simulink model "example"  (R2018a)
settings: Solver=FixedStepAuto  StartTime=0.0  StopTime=data.T_end  FixedStep=1e-4  RelTol=1e-3
InitFcn:
  | run initSim
StopFcn:
  | run endSim
undefined symbols (not defined in the file or in its folder): data
libraries: simulink x2
settings Model: Creator=Matteo Ragni  LastModifiedBy=nirva

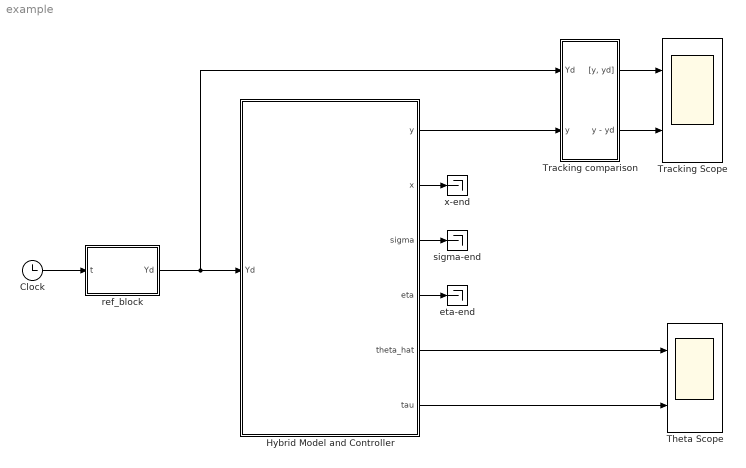
== system example ==
  Clock : Clock
  Hybrid Model and Controller : Subsystem
  Theta Scope : Scope  NumInputPorts=2
  Tracking Scope : Scope  NumInputPorts=2
  Tracking comparison : Subsystem
  eta-end : Terminator
  ref_block : MATLAB Function  TreatAsAtomicUnit=on
  sigma-end : Terminator
  x-end : Terminator
  wires:
  Clock/1 -> ref_block/1(t)
  ref_block/1(Yd) -> Tracking comparison/1(Yd), Hybrid Model and Controller/1(Yd)
  Hybrid Model and Controller/1(y) -> Tracking comparison/2(y)
  Tracking comparison/1("[y, yd]") -> Tracking Scope/1
  Tracking comparison/2(y - yd) -> Tracking Scope/2
  Hybrid Model and Controller/2(x) -> x-end/1
  Hybrid Model and Controller/3(sigma) -> sigma-end/1
  Hybrid Model and Controller/4(eta) -> eta-end/1
  Hybrid Model and Controller/5(theta_hat) -> Theta Scope/1
  Hybrid Model and Controller/6(tau) -> Theta Scope/2

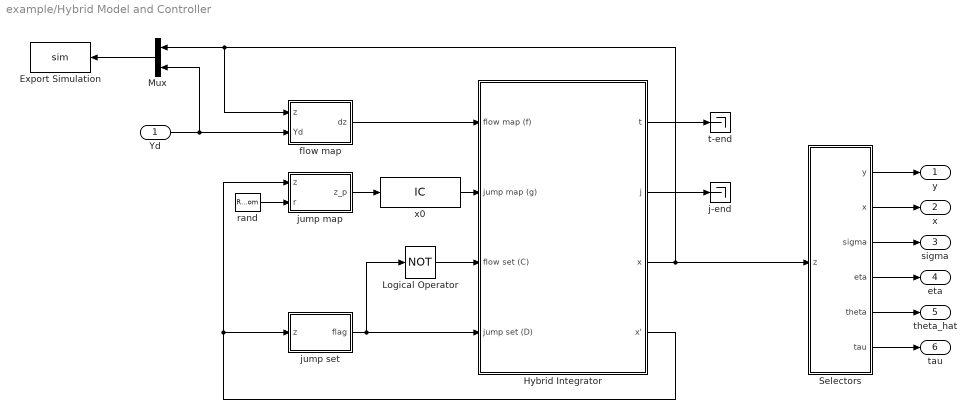
== system example/Hybrid Model and Controller ==
  Yd : Inport
  Export Simulation : ToWorkspace  VariableName=sim  SampleTime=-1
  Hybrid Integrator : Subsystem
  Logical Operator : Logic  Operator=NOT  AllPortsSameDT=off  OutDataTypeStr=boolean
  Mux : Mux  Inputs=2
  Selectors : Subsystem
  flow map : MATLAB Function  TreatAsAtomicUnit=on
  j-end : Terminator
  jump map : MATLAB Function  Priority=2  TreatAsAtomicUnit=on
  jump set : MATLAB Function  TreatAsAtomicUnit=on
  rand : UniformRandomNumber  Minimum=0  SampleTime=0.001
  t-end : Terminator
  x0 : InitialCondition  Value=data.ics
  y : Outport
  x : Outport  Port=2
  sigma : Outport  Port=3
  eta : Outport  Port=4
  theta_hat : Outport  Port=5
  tau : Outport  Port=6
  wires:
  Yd/1 -> Mux/2, flow map/2(Yd)
  Hybrid Integrator/1(t) -> t-end/1
  Hybrid Integrator/2(j) -> j-end/1
  Hybrid Integrator/4(x') -> jump map/1(z), jump set/1(z)
  jump set/1(flag) -> Hybrid Integrator/4(jump set (D)), Logical Operator/1
  Hybrid Integrator/3(x) -> Selectors/1(z), flow map/1(z), Mux/1
  flow map/1(dz) -> Hybrid Integrator/1(flow map (f))
  jump map/1(z_p) -> x0/1
  x0/1 -> Hybrid Integrator/2(jump map (g))
  Logical Operator/1 -> Hybrid Integrator/3(flow set (C))
  rand/1 -> jump map/2(r)
  Selectors/1(y) -> y/1
  Selectors/2(x) -> x/1
  Selectors/3(sigma) -> sigma/1
  Selectors/4(eta) -> eta/1
  Selectors/5(theta) -> theta_hat/1
  Selectors/6(tau) -> tau/1
  Mux/1 -> Export Simulation/1

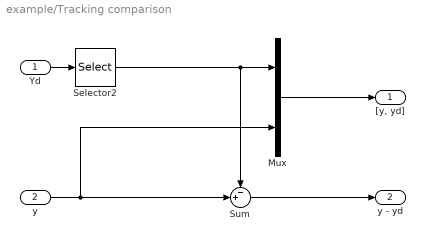
== system example/Tracking comparison ==
  Yd : Inport
  y : Inport  Port=2
  Mux : Mux  Inputs=2
  Selector2 : Selector  InputPortWidth=data.theta_n  IndexOptions=Index vector (dialog)  Indices=[1]  OutputSizes=1
  Sum : Sum  Inputs=-+|
  "[y, yd]" : Outport
  y - yd : Outport  Port=2
  wires:
  Yd/1 -> Selector2/1
  Selector2/1 -> Sum/1, Mux/1
  Mux/1 -> "[y, yd]"/1
  Sum/1 -> y - yd/1
  y/1 -> Mux/2, Sum/2

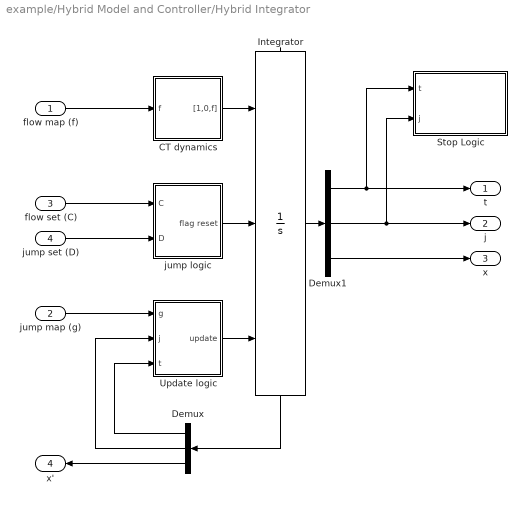
== system example/Hybrid Model and Controller/Hybrid Integrator ==
  flow map (f) : Inport
  jump map (g) : Inport  Port=2
  flow set (C) : Inport  Port=3
  jump set (D) : Inport  Port=4
  CT dynamics : Subsystem
  Demux : Demux  Outputs=[1 ,1, length(data.ics)]
  Demux1 : Demux  Outputs=[1, 1, length(data.ics)]
  Integrator : Integrator  ExternalReset=level hold  InitialConditionSource=external  ShowStatePort=on  ZeroCross=off
  Stop Logic : Subsystem
  Update logic : Subsystem
  jump logic : Subsystem
  t : Outport
  j : Outport  Port=2
  x : Outport  Port=3
  x' : Outport  Port=4
  wires:
  Integrator/State -> Demux/1
  flow map (f)/1 -> CT dynamics/1(f)
  flow set (C)/1 -> jump logic/1(C)
  CT dynamics/1("[1,0,f]") -> Integrator/1
  jump logic/1(flag reset) -> Integrator/2
  jump set (D)/1 -> jump logic/2(D)
  Update logic/1(update) -> Integrator/3
  Demux/1 -> Update logic/3(t)
  Demux/2 -> Update logic/2(j)
  jump map (g)/1 -> Update logic/1(g)
  Demux/3 -> x'/1
  Integrator/1 -> Demux1/1
  Demux1/1 -> Stop Logic/1(t), t/1
  Demux1/2 -> Stop Logic/2(j), j/1
  Demux1/3 -> x/1

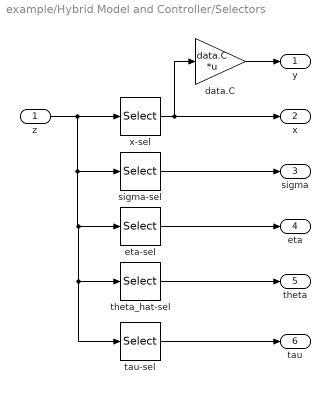
== system example/Hybrid Model and Controller/Selectors ==
  z : Inport
  data.C : Gain  Gain=data.C  Multiplication=Matrix(K*u)
  eta-sel : Selector  InputPortWidth=size(data.ics, 1)  IndexOptions=Index vector (dialog)  Indices=data.index.eta  OutputSizes=1
  sigma-sel : Selector  InputPortWidth=size(data.ics, 1)  IndexOptions=Index vector (dialog)  Indices=data.index.sigma  OutputSizes=1
  tau-sel : Selector  InputPortWidth=size(data.ics, 1)  IndexOptions=Index vector (dialog)  Indices=data.index.tau  OutputSizes=1
  theta_hat-sel : Selector  InputPortWidth=size(data.ics, 1)  IndexOptions=Index vector (dialog)  Indices=data.index.theta_hat  OutputSizes=1
  x-sel : Selector  InputPortWidth=size(data.ics, 1)  IndexOptions=Index vector (dialog)  Indices=data.index.x  OutputSizes=1
  y : Outport
  x : Outport  Port=2
  sigma : Outport  Port=3
  eta : Outport  Port=4
  theta : Outport  Port=5
  tau : Outport  Port=6
  wires:
  z/1 -> tau-sel/1, theta_hat-sel/1, eta-sel/1, sigma-sel/1, x-sel/1
  x-sel/1 -> x/1, data.C/1
  sigma-sel/1 -> sigma/1
  theta_hat-sel/1 -> theta/1
  data.C/1 -> y/1
  tau-sel/1 -> tau/1
  eta-sel/1 -> eta/1

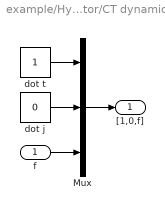
== system example/Hybrid Model and Controller/Hybrid Integrator/CT dynamics ==
  f : Inport
  Mux : Mux  Inputs=3
  dot j : Constant  Value=0
  dot t : Constant
  "[1,0,f]" : Outport
  wires:
  Mux/1 -> "[1,0,f]"/1
  f/1 -> Mux/3
  dot t/1 -> Mux/1
  dot j/1 -> Mux/2

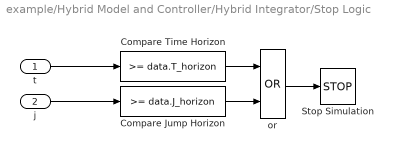
== system example/Hybrid Model and Controller/Hybrid Integrator/Stop Logic ==
  t : Inport
  j : Inport  Port=2
  Compare Jump Horizon : simulink/Logic and Bit Operations/Compare To Constant  relop=>=  const=data.J_horizon  OutDataTypeStr=boolean
  Compare Time Horizon : simulink/Logic and Bit Operations/Compare To Constant  relop=>=  const=data.T_horizon  OutDataTypeStr=boolean
  Stop Simulation : Stop
  or : Logic  Operator=OR  AllPortsSameDT=off  OutDataTypeStr=boolean
  wires:
  Compare Jump Horizon/1 -> or/2
  t/1 -> Compare Time Horizon/1
  j/1 -> Compare Jump Horizon/1
  Compare Time Horizon/1 -> or/1
  or/1 -> Stop Simulation/1

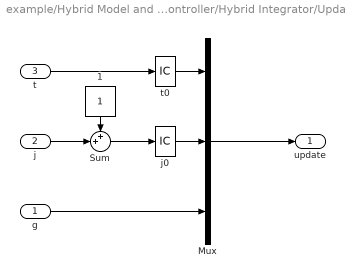
== system example/Hybrid Model and Controller/Hybrid Integrator/Update logic ==
  g : Inport
  j : Inport  Port=2
  t : Inport  Port=3
  1 : Constant
  Mux : Mux  Inputs=3
  Sum : Sum  Inputs=++|
  j0 : InitialCondition  Value=0
  t0 : InitialCondition  Value=0
  update : Outport
  wires:
  Mux/1 -> update/1
  t/1 -> t0/1
  g/1 -> Mux/3
  1/1 -> Sum/1
  j/1 -> Sum/2
  t0/1 -> Mux/1
  Sum/1 -> j0/1
  j0/1 -> Mux/2

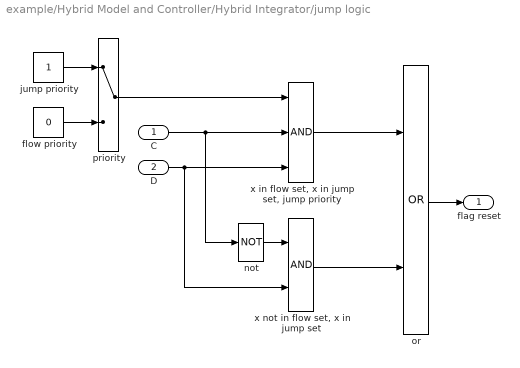
== system example/Hybrid Model and Controller/Hybrid Integrator/jump logic ==
  C : Inport
  D : Inport  Port=2
  flow priority : Constant  Value=0
  jump priority : Constant
  not : Logic  Operator=NOT  Inputs=3  AllPortsSameDT=off  OutDataTypeStr=boolean
  or : Logic  Operator=OR  AllPortsSameDT=off  OutDataTypeStr=boolean
  priority : ManualSwitch
  "x in flow set, x in jump set, jump priority" : Logic  Inputs=3  AllPortsSameDT=off  OutDataTypeStr=boolean
  "x not in flow set, x in jump set" : Logic  AllPortsSameDT=off  OutDataTypeStr=boolean
  flag reset : Outport
  wires:
  jump priority/1 -> priority/1
  flow priority/1 -> priority/2
  D/1 -> "x in flow set, x in jump set, jump priority"/3, "x not in flow set, x in jump set"/2
  C/1 -> not/1, "x in flow set, x in jump set, jump priority"/2
  priority/1 -> "x in flow set, x in jump set, jump priority"/1
  not/1 -> "x not in flow set, x in jump set"/1
  "x in flow set, x in jump set, jump priority"/1 -> or/1
  "x not in flow set, x in jump set"/1 -> or/2
  or/1 -> flag reset/1

== matlab function example/ref_block ==
  data: t input; Yd output
function Yd = ref_block(t)
%#codegen

%    This function was generated by the Symbolic Math Toolbox version 8.1.
%    21-Sep-2018 11:48:09

t2 = t.*(2.0./5.0);
t3 = t.*(1.0./5.0);
t4 = pi.*(1.0./3.0);
t5 = t+t4;
t6 = cos(t3);
t7 = sin(t2);
t8 = cos(t5);
Yd = [t6.*5.0+t7+t8;cos(t2).*(2.0./5.0)-sin(t3)-sin(t5);t6.*(-1.0./5.0)-t7.*(4.0./2.5e1)-t8];

== matlab function example/Hybrid Model and Controller/flow map ==
  data: z input; dz output; Yd input; data parameter
function dz = f(z, Yd, data)
  dz = zeros(size(data.ics));  
  
  %% Signal selection
  x          = z(data.index.x);
  sigma      = z(data.index.sigma);
  eta        = z(data.index.eta);
  theta_hat  = z(data.index.theta_hat);
  
  %% Feed Forward evaluation
  u_ff       = theta_hat' * Yd;
  
  %% Model 
  dx         = data.A * x + data.B * u_ff;
  
  %% Controller
  dsigma     = data.Lambda * sigma + data.Phi * data.C * x;
  deta       = data.Lambda * eta + data.Phi * u_ff;
  dtheta_hat = zeros(data.theta_n, 1);
  dtau       = 1;
  
  %% Out
  dz = [ dx; dsigma; deta; dtheta_hat; dtau; 0];
end

== matlab function example/Hybrid Model and Controller/jump map ==
  data: z input; z_p output; r input; data parameter
function z_p = g(z, r, data)
  z_p = zeros(size(data.ics));  


  %% Signal Selection
  x          = z(data.index.x);
  sigma      = z(data.index.sigma);
  eta        = z(data.index.eta);
  theta_hat  = z(data.index.theta_hat);
  
  e1         = [1; 0; 0];
  
  %% Model
  x_p         = x;
  
  %% Controller
  sigma_p     = sigma;
  eta_p       = sigma;
  theta_hat_p = theta_hat - data.gamma * sigma /(max(sigma' * sigma, data.epsilon^2)) * (sigma' * theta_hat - e1' * eta);
  tau_p       = 0;
  
  %% Random selection for next trigger
  tau_set_p   = data.tau_min + (data.tau_max - data.tau_min) * r;
  
  %% Output
  z_p = [ x_p; sigma_p; eta_p; theta_hat_p; tau_p; tau_set_p];
  
end

== matlab function example/Hybrid Model and Controller/jump set ==
  data: z input; flag output; data parameter
function flag  = D(z, data) 
  
  tau     = z(data.index.tau);
  tau_set = z(data.index.tau_set);
  
  flag = 0;
  if (tau >= tau_set)
    flag = 1;
  end
  
end
